simulink library "LiS_ECN_Model_lib"  (R2016a)
settings: Solver=ode45  StartTime=0.0  StopTime=10.0  RelTol=1e-3
undefined symbols (not defined in the file): C1_SOC_POLY20, C1_SOC_POLY30, C1_SOC_POLY50, C_man, Cap_all, DiscIntNeverNeededParam, OCV_POLYhigh20, OCV_POLYhigh30, OCV_POLYhigh50, OCV_POLYlow20, OCV_POLYlow30, OCV_POLYlow50, R1_SOC_POLY20, R1_SOC_POLY30, R1_SOC_POLY50, Ri_POLYhigh20, Ri_POLYhigh30, Ri_POLYhigh50, Ri_POLYlow20, Ri_POLYlow30, Ri_POLYlow50, StrechFactors, T, Tempstrech
libraries: simulink x1
settings Model: Creator=e102261  LastModifiedBy=e102261
settings DataIOCC: LimitDataPoints=on
settings DebuggingCC: AllowSymbolicDim=off

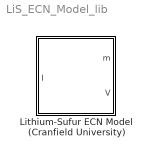
== system LiS_ECN_Model_lib ==
  Lithium-Sufur ECN Model (Cranfield University) : Subsystem  mask(Lithium-Sulfur ECN Model (Cranfield University)){TempDegC=21, InitialSoC=1, Ts=1}
      mask prompts: TempDegC "Temperature (degrees C):"; InitialSoC "Initial State-of-Charge (normalized):"; Ts "Sample time (-1 for inherited):"
      mask help:
      | This block contains an Equivalent Circuit (ECN) model of a representative lithium-sulfur cell supplied by OXIS Energy.  The model was developed as part of the Revolutionary Electric Vehicle Battery (REVB) project co-funded by Innovate UK, and contributions were made by people at Cranfield University, Imperial College London and OXIS Energy.
      |
      | This model is released in association with a the paper 'Multi-temperature state-dependent equivalent circuit discharge model for lithium-sulfur batteries' by Propp et al, accepted by the Journal of Power Sources on July 23, 2016, http://dx.doi.org/10.1016/j.jpowsour.2016.07.090.  Please reference this paper if you use this model.
      |
      | Please see the licence terms at http://dx.doi.org/10.17862/cranfield.rd.c.3292031
      mask init:
      | % Define the MATLAB data file.
      | MATLAB_DATA_FILE = 'LiS_ECN_Model_Parameters.mat';
      | 
      | % Check to see if the file exists: if not, fail gracefully.
      | fileExists = exist(MATLAB_DATA_FILE, 'file') > 0;
      | if ~fileExists
      |     id = 'LiS_ECN_Model:parameterFileNotFound';
      |     msg = {'Parameter file not found: %s.', MATLAB_DATA_FILE};
      |     ME = MException(id, msg{:});
      |     throw(ME);
      | end
      | 
      | % If the file does exist, then load it into the block
      | % workspace.
      | load(MATLAB_DATA_FILE);
      | 
      | try
      |     theImage = imread('oxiscellicon_simulink')
      | catch
      |     theImage = [];
      | end
      settings: AttributesFormatString=|
      | Temperature = %<TempDegC> deg C
      | Initial SoC = %<InitialSoC>
      mask Display:
      | patch([0 0 1 1],[0 1 1 0],[255 221 0]/255);
      | image(imread('oxis_li-s.png'),'center')
      | plot([0.5 0.5], [0.05 0.40]);
      | plot([0.35 0.35 0.65 0.65 0.35], [0.45 0.4 0.4 0.45 0.45]);
      | %patch([0.35 0.35 0.65 0.65 0.35], [0.45 0.4 0.4 0.45 0.45]);
      | plot([0.2 0.8], [0.55 0.55]);
      | plot([0.5 0.5], [0.55 0.95]);
      | 
      | port_label('output', 1, 'm')
      | color('blue')
      | port_label('input', 1, 'I(t)')
      | port_label('output', 2, 'V(t)')

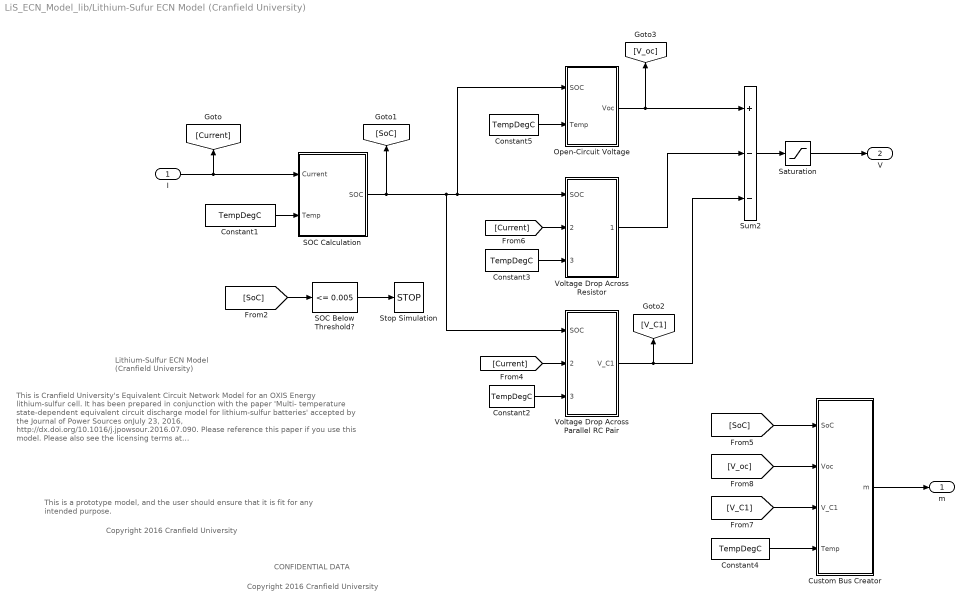
== system LiS_ECN_Model_lib/Lithium-Sufur ECN Model (Cranfield University) ==
  note: Copyright 2016 Cranfield University
  note: CONFIDENTIAL DATA
  note: Copyright 2016 Cranfield University
  note: This is Cranfield University's Equivalent Circuit Network Model for an OXIS Energy
      | lithium-sulfur cell. It has been prepared in conjunction with the paper 'Multi-
      | temperature state-dependent equivalent circuit discharge model for lithium-sulfur
      | batteries' accepted by the Journal of Power Sources onJuly 23, 2016,
      | http://dx.doi.org/10.1016/j.jpowsour.2016.07.090. Please reference this paper if
      | you use this model.
      |
      | Please also see the licensing terms at
      | http://dx.doi.org/10.17862/cranfield.rd.c.3292031
  note: Lithium-Sulfur ECN Model
      | (Cranfield University)
  note: This is a prototype model, and the user should ensure that it is fit for
      | any intended purpose.
  I : Inport  PortDimensions=1  SampleTime=Ts
      settings: AttributesFormatString=SampleTime=%<SampleTime>
  Constant{1..5} (5 alike) : Constant  Value=TempDegC
  Custom Bus Creator : Subsystem
  Open-Circuit Voltage : Subsystem
  SOC Below Threshold? : simulink/Logic and Bit Operations/Compare To Constant  relop=<=  const=0.005  OutDataTypeStr=boolean
  SOC Calculation : Subsystem
  Saturation : Saturate  UpperLimit=inf  LowerLimit=0
      settings: AttributesFormatString=|
      | UpperLimit=%<UpperLimit>
      | LowerLimit=%<LowerLimit>
  Stop Simulation : Stop
  Sum2 : Sum  Inputs=+--
  Voltage Drop Across Parallel RC Pair : Subsystem
  Voltage Drop Across Resistor : Subsystem
  m : Outport  SampleTime=Ts
      settings: AttributesFormatString=SampleTime=%<SampleTime>
  V : Outport  Port=2  SampleTime=Ts
      settings: AttributesFormatString=SampleTime=%<SampleTime>
  wires:
  Custom Bus Creator/1(m) -> m/1
  Constant4/1 -> Custom Bus Creator/4(Temp)
  [V_C1] -> Custom Bus Creator/3(V_C1)
  [V_oc] -> Custom Bus Creator/2(Voc)
  [SoC] -> Custom Bus Creator/1(SoC)
  SOC Below Threshold?/1 -> Stop Simulation/1
  Constant1/1 -> SOC Calculation/2(Temp)
  Constant2/1 -> Voltage Drop Across Parallel RC Pair/3(Temperature)
  Constant3/1 -> Voltage Drop Across Resistor/3(Temp)
  Constant5/1 -> Open-Circuit Voltage/2(Temp)
  Saturation/1 -> V/1
  SOC Calculation/1(SOC) -> [SoC], Voltage Drop Across Parallel RC Pair/1(SOC), Voltage Drop Across Resistor/1(SOC), Open-Circuit Voltage/1(SOC)
  [Current] -> Voltage Drop Across Parallel RC Pair/2(Current)
  Voltage Drop Across Parallel RC Pair/1(V_C1) -> [V_C1], Sum2/3
  Voltage Drop Across Resistor/1(V Rint) -> Sum2/2
  [Current] -> Voltage Drop Across Resistor/2(Current)
  Open-Circuit Voltage/1(Voc) -> [V_oc], Sum2/1
  [SoC] -> SOC Below Threshold?/1
  I/1 -> [Current], SOC Calculation/1(Current)
  Sum2/1 -> Saturation/1

== system LiS_ECN_Model_lib/Lithium-Sufur ECN Model (Cranfield University)/Custom Bus Creator ==
  SoC : Inport  PortDimensions=1  SampleTime=Ts
  Voc : Inport  Port=2  PortDimensions=1  SampleTime=Ts
  V_C1 : Inport  Port=3  PortDimensions=1  SampleTime=Ts
  Temp : Inport  Port=4  PortDimensions=1  SampleTime=Ts
  Bus Creator : BusCreator  Inputs=4
  m : Outport
  wires:
  Bus Creator/1 -> m/1
  Temp/1 -> Bus Creator/4  "Temperature (deg C)"
  V_C1/1 -> Bus Creator/3  "Voltage across C1 (V)"
  Voc/1 -> Bus Creator/2  "Open-circuit voltage (V)"
  SoC/1 -> Bus Creator/1  "State-of-Charge (dimensionless)"

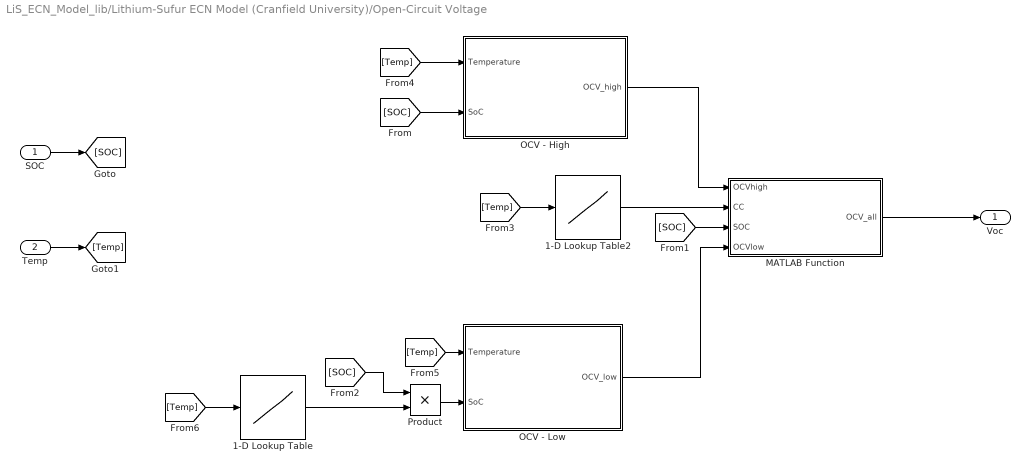
== system LiS_ECN_Model_lib/Lithium-Sufur ECN Model (Cranfield University)/Open-Circuit Voltage ==
  SOC : Inport
  Temp : Inport  Port=2
  1-D Lookup Table : Lookup_n-D  NumberOfTableDimensions=1  BreakpointsForDimension1=Tempstrech  Table=StrechFactors  InternalRulePriority=Speed  RndMeth=Simplest  InputSameDT=on
  1-D Lookup Table2 : Lookup_n-D  NumberOfTableDimensions=1  BreakpointsForDimension1=Temp'  Table=C_man  InternalRulePriority=Speed  RndMeth=Simplest  InputSameDT=on
  MATLAB Function : MATLAB Function  TreatAsAtomicUnit=on
  OCV - High : Subsystem
  OCV - Low : Subsystem
  Product : Product
  Voc : Outport
  wires:
  1-D Lookup Table2/1 -> MATLAB Function/2(CC)
  OCV - High/1("OCV_high ") -> MATLAB Function/1(OCVhigh)
  SOC/1 -> [SOC]
  [SOC] -> OCV - High/2(SoC)
  [SOC] -> MATLAB Function/3(SOC)
  [Temp] -> OCV - High/1(Temperature)
  [Temp] -> 1-D Lookup Table2/1
  [SOC] -> Product/1
  Temp/1 -> [Temp]
  [Temp] -> OCV - Low/1(Temperature)
  MATLAB Function/1(OCV_all) -> Voc/1
  [Temp] -> 1-D Lookup Table/1
  1-D Lookup Table/1 -> Product/2
  Product/1 -> OCV - Low/2(SoC)
  OCV - Low/1("OCV_low ") -> MATLAB Function/4(OCVlow)

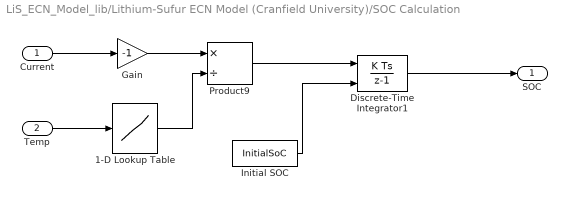
== system LiS_ECN_Model_lib/Lithium-Sufur ECN Model (Cranfield University)/SOC Calculation ==
  Current : Inport
  Temp : Inport  Port=2
  1-D Lookup Table : Lookup_n-D  NumberOfTableDimensions=1  BreakpointsForDimension1=T  Table=Cap_all  InternalRulePriority=Speed  RndMeth=Simplest  InputSameDT=on
  Discrete-Time Integrator1 : DiscreteIntegrator  InitialConditionSource=external  InitialConditionSetting=State (most efficient)  SampleTime=Ts  ICPrevOutput=DiscIntNeverNeededParam  ICPrevScaledInput=DiscIntNeverNeededParam
  Gain : Gain  Gain=-1
  Initial SOC : Constant  Value=InitialSoC
  Product9 : Product  Inputs=*/
  SOC : Outport
  wires:
  Initial SOC/1 -> Discrete-Time Integrator1/2
  Discrete-Time Integrator1/1 -> SOC/1
  1-D Lookup Table/1 -> Product9/2
  Temp/1 -> 1-D Lookup Table/1
  Product9/1 -> Discrete-Time Integrator1/1
  Gain/1 -> Product9/1
  Current/1 -> Gain/1

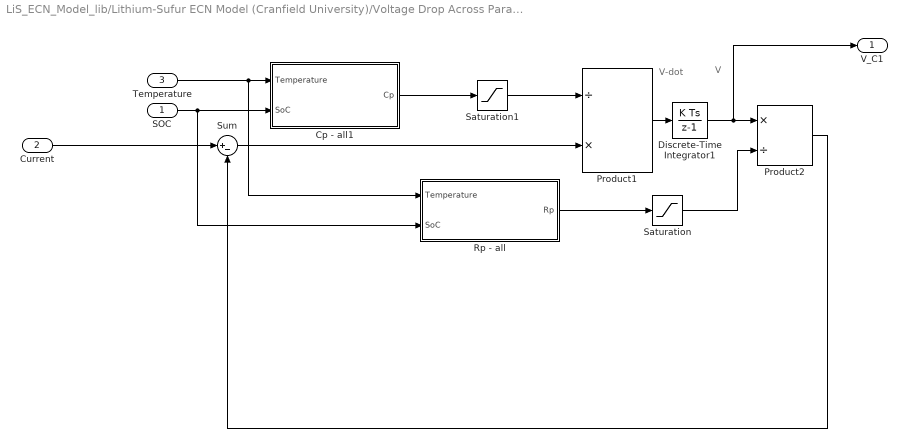
== system LiS_ECN_Model_lib/Lithium-Sufur ECN Model (Cranfield University)/Voltage Drop Across Parallel RC Pair ==
  note: V-dot
  note: V
  SOC : Inport
  Current : Inport  Port=2
  Temperature : Inport  Port=3
  Cp - all1 : Subsystem
  Discrete-Time Integrator1 : DiscreteIntegrator  SampleTime=Ts  ICPrevOutput=DiscIntNeverNeededParam  ICPrevScaledInput=DiscIntNeverNeededParam
  Product1 : Product  Inputs=/*
  Product2 : Product  Inputs=*/
  Rp - all : Subsystem
  Saturation : Saturate  UpperLimit=inf  LowerLimit=0.0001
  Saturation1 : Saturate  UpperLimit=50000  LowerLimit=10
  Sum : Sum  Inputs=|+-
  V_C1 : Outport
  wires:
  Temperature/1 -> Cp - all1/1(Temperature), Rp - all/1(Temperature)
  Cp - all1/1("Cp ") -> Saturation1/1
  Rp - all/1("Rp ") -> Saturation/1
  Product2/1 -> Sum/2
  Discrete-Time Integrator1/1 -> Product2/1, V_C1/1
  Saturation/1 -> Product2/2
  Product1/1 -> Discrete-Time Integrator1/1
  Sum/1 -> Product1/2
  Saturation1/1 -> Product1/1
  Current/1 -> Sum/1
  SOC/1 -> Cp - all1/2(SoC), Rp - all/2(SoC)

== system LiS_ECN_Model_lib/Lithium-Sufur ECN Model (Cranfield University)/Voltage Drop Across Resistor ==
  SOC : Inport
  Current : Inport  Port=2
  Temp : Inport  Port=3
  Product : Product
  Ri - All : Subsystem
  V Rint : Outport
  wires:
  Ri - All/1(Ri all) -> Product/1
  Temp/1 -> Ri - All/2(Temp1)
  SOC/1 -> Ri - All/1(SoC)
  Product/1 -> V Rint/1
  Current/1 -> Product/2

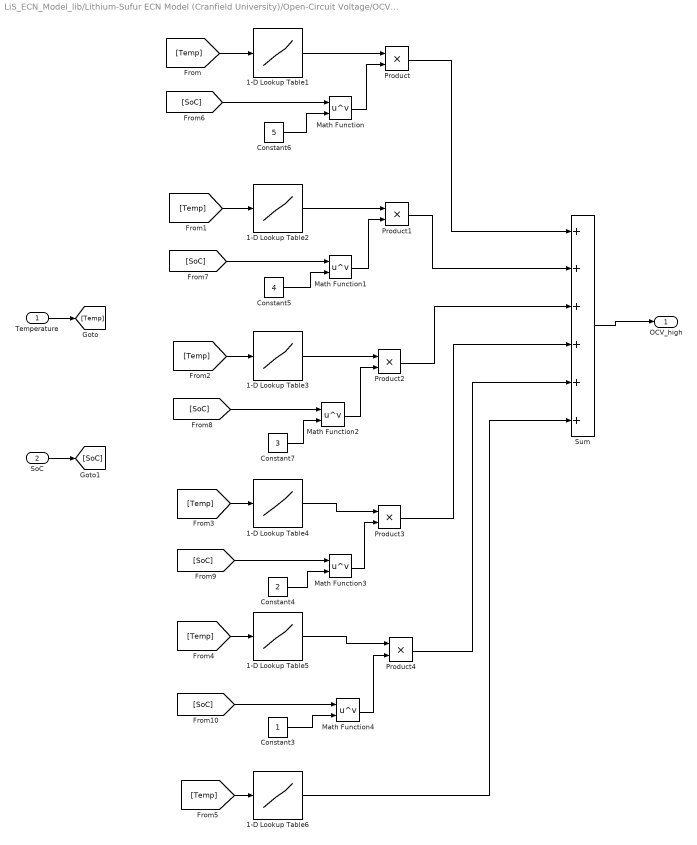
== system LiS_ECN_Model_lib/Lithium-Sufur ECN Model (Cranfield University)/Open-Circuit Voltage/OCV - High ==
  Temperature : Inport
  SoC : Inport  Port=2
  1-D Lookup Table1 : Lookup_n-D  NumberOfTableDimensions=1  BreakpointsForDimension1=T  Table=[OCV_POLYhigh20(1) ; OCV_POLYhigh30(1) ; OCV_POLYhigh50(1)]  InternalRulePriority=Speed  RndMeth=Simplest  InputSameDT=on
  1-D Lookup Table2 : Lookup_n-D  NumberOfTableDimensions=1  BreakpointsForDimension1=T  Table=[OCV_POLYhigh20(2) ; OCV_POLYhigh30(2) ; OCV_POLYhigh50(2)]  InternalRulePriority=Speed  RndMeth=Simplest  InputSameDT=on
  1-D Lookup Table3 : Lookup_n-D  NumberOfTableDimensions=1  BreakpointsForDimension1=T  Table=[OCV_POLYhigh20(3) ; OCV_POLYhigh30(3) ; OCV_POLYhigh50(3)]  InternalRulePriority=Speed  RndMeth=Simplest  InputSameDT=on
  1-D Lookup Table4 : Lookup_n-D  NumberOfTableDimensions=1  BreakpointsForDimension1=T  Table=[OCV_POLYhigh20(4) ; OCV_POLYhigh30(4) ; OCV_POLYhigh50(4)]  InternalRulePriority=Speed  RndMeth=Simplest  InputSameDT=on
  1-D Lookup Table5 : Lookup_n-D  NumberOfTableDimensions=1  BreakpointsForDimension1=T  Table=[OCV_POLYhigh20(5) ; OCV_POLYhigh30(5) ; OCV_POLYhigh50(5)]  InternalRulePriority=Speed  RndMeth=Simplest  InputSameDT=on
  1-D Lookup Table6 : Lookup_n-D  NumberOfTableDimensions=1  BreakpointsForDimension1=T  Table=[OCV_POLYhigh20(6) ; OCV_POLYhigh30(6) ; OCV_POLYhigh50(6)]  InternalRulePriority=Speed  RndMeth=Simplest  InputSameDT=on
  Constant3 : Constant
  Constant4 : Constant  Value=2
  Constant5 : Constant  Value=4
  Constant6 : Constant  Value=5
  Constant7 : Constant  Value=3
  Math Function{,1..4} (5 alike) : Math  Operator=pow  SaturateOnIntegerOverflow=on
  Product{,1..4} (5 alike) : Product
  Sum : Sum  Inputs=++++++
  "OCV_high " : Outport
  wires:
  SoC/1 -> [SoC]
  Constant6/1 -> Math Function/2
  Math Function4/1 -> Product4/2
  1-D Lookup Table4/1 -> Product3/1
  Math Function3/1 -> Product3/2
  Constant4/1 -> Math Function3/2
  Product2/1 -> Sum/3
  Product4/1 -> Sum/5
  1-D Lookup Table5/1 -> Product4/1
  Math Function2/1 -> Product2/2
  Product/1 -> Sum/1
  Constant7/1 -> Math Function2/2
  Product3/1 -> Sum/4
  Constant5/1 -> Math Function1/2
  1-D Lookup Table2/1 -> Product1/1
  Constant3/1 -> Math Function4/2
  1-D Lookup Table3/1 -> Product2/1
  1-D Lookup Table6/1 -> Sum/6
  Product1/1 -> Sum/2
  Math Function1/1 -> Product1/2
  1-D Lookup Table1/1 -> Product/1
  Math Function/1 -> Product/2
  [Temp] -> 1-D Lookup Table5/1
  [Temp] -> 1-D Lookup Table6/1
  [Temp] -> 1-D Lookup Table4/1
  [SoC] -> Math Function/1
  [SoC] -> Math Function2/1
  [SoC] -> Math Function4/1
  [SoC] -> Math Function3/1
  [SoC] -> Math Function1/1
  Temperature/1 -> [Temp]
  [Temp] -> 1-D Lookup Table1/1
  [Temp] -> 1-D Lookup Table2/1
  [Temp] -> 1-D Lookup Table3/1
  Sum/1 -> "OCV_high "/1

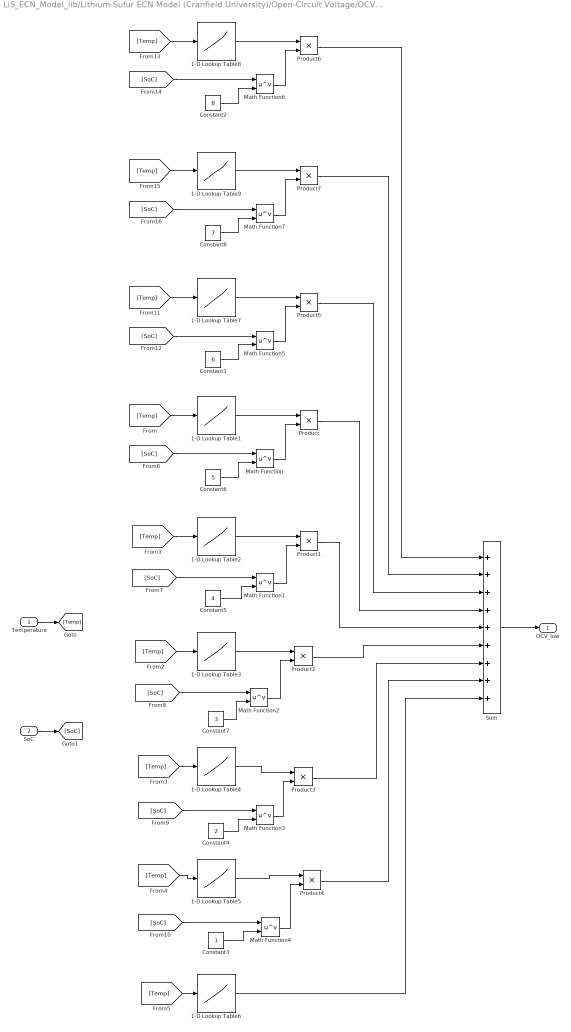
== system LiS_ECN_Model_lib/Lithium-Sufur ECN Model (Cranfield University)/Open-Circuit Voltage/OCV - Low ==
  Temperature : Inport
  SoC : Inport  Port=2
  1-D Lookup Table1 : Lookup_n-D  NumberOfTableDimensions=1  BreakpointsForDimension1=T  Table=[OCV_POLYlow20(4) ; OCV_POLYlow30(4) ; OCV_POLYlow50(4)]  InternalRulePriority=Speed  RndMeth=Simplest  InputSameDT=on
  1-D Lookup Table2 : Lookup_n-D  NumberOfTableDimensions=1  BreakpointsForDimension1=T  Table=[OCV_POLYlow20(5) ; OCV_POLYlow30(5) ; OCV_POLYlow50(5)]  InternalRulePriority=Speed  RndMeth=Simplest  InputSameDT=on
  1-D Lookup Table3 : Lookup_n-D  NumberOfTableDimensions=1  BreakpointsForDimension1=T  Table=[OCV_POLYlow20(6) ; OCV_POLYlow30(6) ; OCV_POLYlow50(6)]  InternalRulePriority=Speed  RndMeth=Simplest  InputSameDT=on
  1-D Lookup Table4 : Lookup_n-D  NumberOfTableDimensions=1  BreakpointsForDimension1=T  Table=[OCV_POLYlow20(7) ; OCV_POLYlow30(7) ; OCV_POLYlow50(7)]  InternalRulePriority=Speed  RndMeth=Simplest  InputSameDT=on
  1-D Lookup Table5 : Lookup_n-D  NumberOfTableDimensions=1  BreakpointsForDimension1=T  Table=[OCV_POLYlow20(8) ; OCV_POLYlow30(8) ; OCV_POLYlow50(8)]  InternalRulePriority=Speed  RndMeth=Simplest  InputSameDT=on
  1-D Lookup Table6 : Lookup_n-D  NumberOfTableDimensions=1  BreakpointsForDimension1=T  Table=[OCV_POLYlow20(9) ; OCV_POLYlow30(9) ; OCV_POLYlow50(9)]  InternalRulePriority=Speed  RndMeth=Simplest  InputSameDT=on
  1-D Lookup Table7 : Lookup_n-D  NumberOfTableDimensions=1  BreakpointsForDimension1=T  Table=[OCV_POLYlow20(3) ; OCV_POLYlow30(3) ; OCV_POLYlow50(3)]  InternalRulePriority=Speed  RndMeth=Simplest  InputSameDT=on
  1-D Lookup Table8 : Lookup_n-D  NumberOfTableDimensions=1  BreakpointsForDimension1=T  Table=[OCV_POLYlow20(1) ; OCV_POLYlow30(1) ; OCV_POLYlow50(1)]  InternalRulePriority=Speed  RndMeth=Simplest  InputSameDT=on
  1-D Lookup Table9 : Lookup_n-D  NumberOfTableDimensions=1  BreakpointsForDimension1=T  Table=[OCV_POLYlow20(2) ; OCV_POLYlow30(2) ; OCV_POLYlow50(2)]  InternalRulePriority=Speed  RndMeth=Simplest  InputSameDT=on
  Constant1 : Constant  Value=6
  Constant2 : Constant  Value=8
  Constant3 : Constant
  Constant4 : Constant  Value=2
  Constant5 : Constant  Value=4
  Constant6 : Constant  Value=5
  Constant7 : Constant  Value=3
  Constant8 : Constant  Value=7
  Math Function{,1..7} (8 alike) : Math  Operator=pow  SaturateOnIntegerOverflow=on
  Product{,1..7} (8 alike) : Product
  Sum : Sum  Inputs=+++++++++
  "OCV_low " : Outport
  wires:
  1-D Lookup Table6/1 -> Sum/9
  Product4/1 -> Sum/8
  Product3/1 -> Sum/7
  Product2/1 -> Sum/6
  Product1/1 -> Sum/5
  Product/1 -> Sum/4
  Product5/1 -> Sum/3
  Product7/1 -> Sum/2
  Product6/1 -> Sum/1
  Constant8/1 -> Math Function7/2
  1-D Lookup Table9/1 -> Product7/1
  Math Function7/1 -> Product7/2
  [SoC] -> Math Function7/1
  [Temp] -> 1-D Lookup Table9/1
  Constant2/1 -> Math Function6/2
  1-D Lookup Table8/1 -> Product6/1
  Math Function6/1 -> Product6/2
  [SoC] -> Math Function6/1
  [Temp] -> 1-D Lookup Table8/1
  Constant1/1 -> Math Function5/2
  1-D Lookup Table7/1 -> Product5/1
  Math Function5/1 -> Product5/2
  [SoC] -> Math Function5/1
  [Temp] -> 1-D Lookup Table7/1
  SoC/1 -> [SoC]
  Constant6/1 -> Math Function/2
  Math Function4/1 -> Product4/2
  1-D Lookup Table4/1 -> Product3/1
  Math Function3/1 -> Product3/2
  Constant4/1 -> Math Function3/2
  1-D Lookup Table5/1 -> Product4/1
  Math Function2/1 -> Product2/2
  Constant7/1 -> Math Function2/2
  Constant5/1 -> Math Function1/2
  1-D Lookup Table2/1 -> Product1/1
  Constant3/1 -> Math Function4/2
  1-D Lookup Table3/1 -> Product2/1
  Math Function1/1 -> Product1/2
  1-D Lookup Table1/1 -> Product/1
  Math Function/1 -> Product/2
  [Temp] -> 1-D Lookup Table5/1
  [Temp] -> 1-D Lookup Table6/1
  [Temp] -> 1-D Lookup Table4/1
  [SoC] -> Math Function/1
  [SoC] -> Math Function2/1
  [SoC] -> Math Function4/1
  [SoC] -> Math Function3/1
  [SoC] -> Math Function1/1
  Temperature/1 -> [Temp]
  [Temp] -> 1-D Lookup Table1/1
  [Temp] -> 1-D Lookup Table2/1
  [Temp] -> 1-D Lookup Table3/1
  Sum/1 -> "OCV_low "/1

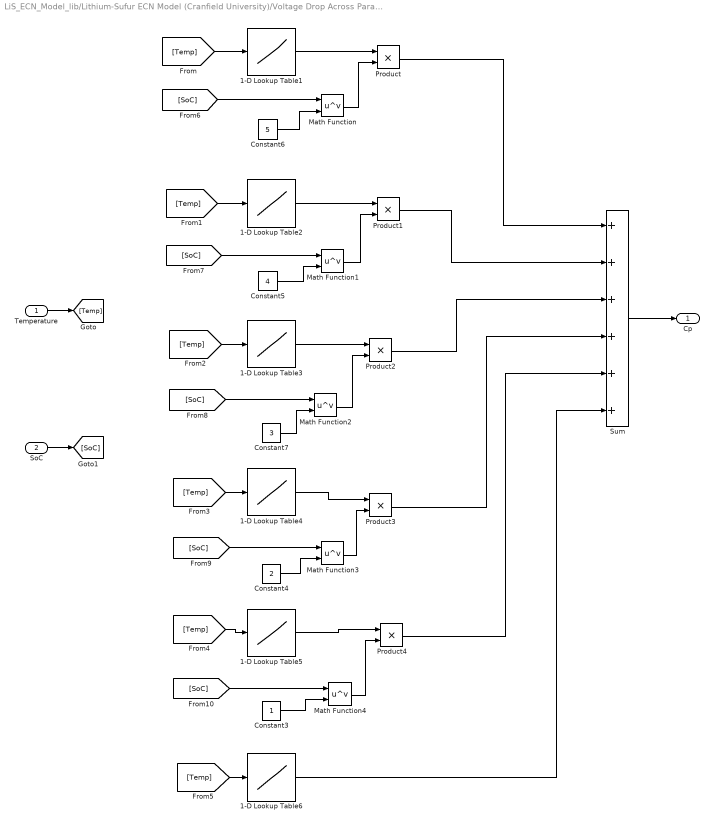
== system LiS_ECN_Model_lib/Lithium-Sufur ECN Model (Cranfield University)/Voltage Drop Across Parallel RC Pair/Cp - all1 ==
  Temperature : Inport
  SoC : Inport  Port=2
  1-D Lookup Table1 : Lookup_n-D  NumberOfTableDimensions=1  BreakpointsForDimension1=T  Table=[C1_SOC_POLY20(1) ; C1_SOC_POLY30(1) ; C1_SOC_POLY50(1)]  InternalRulePriority=Speed  RndMeth=Simplest  InputSameDT=on
  1-D Lookup Table2 : Lookup_n-D  NumberOfTableDimensions=1  BreakpointsForDimension1=T  Table=[C1_SOC_POLY20(2) ; C1_SOC_POLY30(2) ; C1_SOC_POLY50(2)]  InternalRulePriority=Speed  RndMeth=Simplest  InputSameDT=on
  1-D Lookup Table3 : Lookup_n-D  NumberOfTableDimensions=1  BreakpointsForDimension1=T  Table=[C1_SOC_POLY20(3) ; C1_SOC_POLY30(3) ; C1_SOC_POLY50(3)]  InternalRulePriority=Speed  RndMeth=Simplest  InputSameDT=on
  1-D Lookup Table4 : Lookup_n-D  NumberOfTableDimensions=1  BreakpointsForDimension1=T  Table=[C1_SOC_POLY20(4) ; C1_SOC_POLY30(4) ; C1_SOC_POLY50(4)]  InternalRulePriority=Speed  RndMeth=Simplest  InputSameDT=on
  1-D Lookup Table5 : Lookup_n-D  NumberOfTableDimensions=1  BreakpointsForDimension1=T  Table=[C1_SOC_POLY20(5) ; C1_SOC_POLY30(5) ; C1_SOC_POLY50(5)]  InternalRulePriority=Speed  RndMeth=Simplest  InputSameDT=on
  1-D Lookup Table6 : Lookup_n-D  NumberOfTableDimensions=1  BreakpointsForDimension1=T  Table=[C1_SOC_POLY20(6) ; C1_SOC_POLY30(6) ; C1_SOC_POLY50(6)]  InternalRulePriority=Speed  RndMeth=Simplest  InputSameDT=on
  Constant3 : Constant
  Constant4 : Constant  Value=2
  Constant5 : Constant  Value=4
  Constant6 : Constant  Value=5
  Constant7 : Constant  Value=3
  Math Function{,1..4} (5 alike) : Math  Operator=pow  SaturateOnIntegerOverflow=on
  Product{,1..4} (5 alike) : Product
  Sum : Sum  Inputs=++++++
  "Cp " : Outport
  wires:
  1-D Lookup Table6/1 -> Sum/6
  Product4/1 -> Sum/5
  Product3/1 -> Sum/4
  Product2/1 -> Sum/3
  Product1/1 -> Sum/2
  Product/1 -> Sum/1
  SoC/1 -> [SoC]
  Constant6/1 -> Math Function/2
  Math Function4/1 -> Product4/2
  1-D Lookup Table4/1 -> Product3/1
  Math Function3/1 -> Product3/2
  Constant4/1 -> Math Function3/2
  1-D Lookup Table5/1 -> Product4/1
  Math Function2/1 -> Product2/2
  Constant7/1 -> Math Function2/2
  Constant5/1 -> Math Function1/2
  1-D Lookup Table2/1 -> Product1/1
  Constant3/1 -> Math Function4/2
  1-D Lookup Table3/1 -> Product2/1
  Math Function1/1 -> Product1/2
  1-D Lookup Table1/1 -> Product/1
  Math Function/1 -> Product/2
  [Temp] -> 1-D Lookup Table5/1
  [Temp] -> 1-D Lookup Table6/1
  [Temp] -> 1-D Lookup Table4/1
  [SoC] -> Math Function/1
  [SoC] -> Math Function2/1
  [SoC] -> Math Function4/1
  [SoC] -> Math Function3/1
  [SoC] -> Math Function1/1
  Temperature/1 -> [Temp]
  [Temp] -> 1-D Lookup Table1/1
  [Temp] -> 1-D Lookup Table2/1
  [Temp] -> 1-D Lookup Table3/1
  Sum/1 -> "Cp "/1

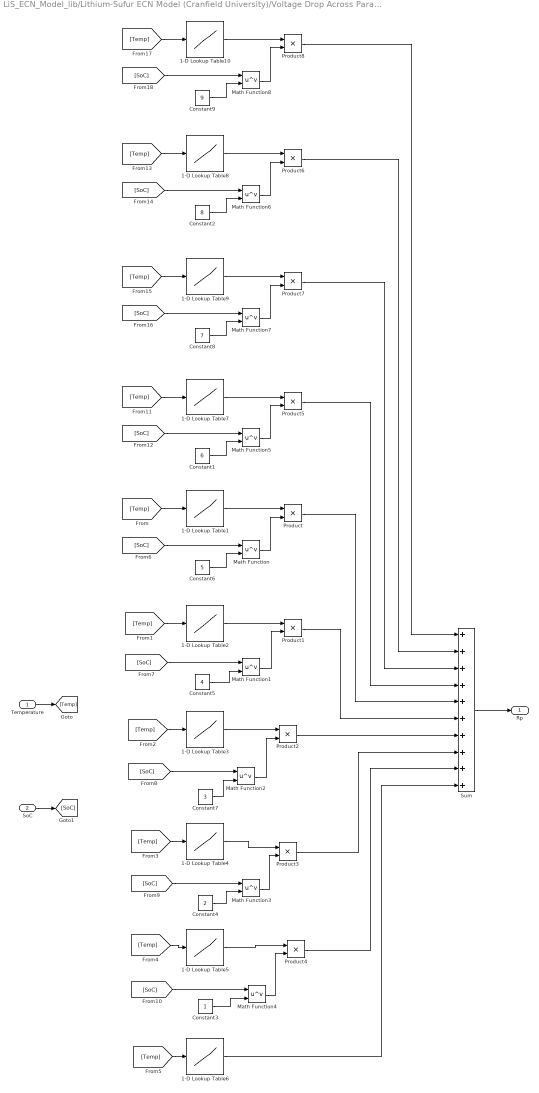
== system LiS_ECN_Model_lib/Lithium-Sufur ECN Model (Cranfield University)/Voltage Drop Across Parallel RC Pair/Rp - all ==
  Temperature : Inport
  SoC : Inport  Port=2
  1-D Lookup Table1 : Lookup_n-D  NumberOfTableDimensions=1  BreakpointsForDimension1=T  Table=[R1_SOC_POLY20(5) ; R1_SOC_POLY30(5) ; R1_SOC_POLY50(5)]  InternalRulePriority=Speed  RndMeth=Simplest  InputSameDT=on
  1-D Lookup Table10 : Lookup_n-D  NumberOfTableDimensions=1  BreakpointsForDimension1=T  Table=[R1_SOC_POLY20(1) ; R1_SOC_POLY30(1) ; R1_SOC_POLY50(1)]  InternalRulePriority=Speed  RndMeth=Simplest  InputSameDT=on
  1-D Lookup Table2 : Lookup_n-D  NumberOfTableDimensions=1  BreakpointsForDimension1=T  Table=[R1_SOC_POLY20(6) ; R1_SOC_POLY30(6) ; R1_SOC_POLY50(6)]  InternalRulePriority=Speed  RndMeth=Simplest  InputSameDT=on
  1-D Lookup Table3 : Lookup_n-D  NumberOfTableDimensions=1  BreakpointsForDimension1=T  Table=[R1_SOC_POLY20(7) ; R1_SOC_POLY30(7) ; R1_SOC_POLY50(7)]  InternalRulePriority=Speed  RndMeth=Simplest  InputSameDT=on
  1-D Lookup Table4 : Lookup_n-D  NumberOfTableDimensions=1  BreakpointsForDimension1=T  Table=[R1_SOC_POLY20(8) ; R1_SOC_POLY30(8) ; R1_SOC_POLY50(8)]  InternalRulePriority=Speed  RndMeth=Simplest  InputSameDT=on
  1-D Lookup Table5 : Lookup_n-D  NumberOfTableDimensions=1  BreakpointsForDimension1=T  Table=[R1_SOC_POLY20(9) ; R1_SOC_POLY30(9) ; R1_SOC_POLY50(9)]  InternalRulePriority=Speed  RndMeth=Simplest  InputSameDT=on
  1-D Lookup Table6 : Lookup_n-D  NumberOfTableDimensions=1  BreakpointsForDimension1=T  Table=[R1_SOC_POLY20(10) ; R1_SOC_POLY30(10) ; R1_SOC_POLY50(10)]  InternalRulePriority=Speed  RndMeth=Simplest  InputSameDT=on
  1-D Lookup Table7 : Lookup_n-D  NumberOfTableDimensions=1  BreakpointsForDimension1=T  Table=[R1_SOC_POLY20(4) ; R1_SOC_POLY30(4) ; R1_SOC_POLY50(4)]  InternalRulePriority=Speed  RndMeth=Simplest  InputSameDT=on
  1-D Lookup Table8 : Lookup_n-D  NumberOfTableDimensions=1  BreakpointsForDimension1=T  Table=[R1_SOC_POLY20(2) ; R1_SOC_POLY30(2) ; R1_SOC_POLY50(2)]  InternalRulePriority=Speed  RndMeth=Simplest  InputSameDT=on
  1-D Lookup Table9 : Lookup_n-D  NumberOfTableDimensions=1  BreakpointsForDimension1=T  Table=[R1_SOC_POLY20(3) ; R1_SOC_POLY30(3) ; R1_SOC_POLY50(3)]  InternalRulePriority=Speed  RndMeth=Simplest  InputSameDT=on
  Constant1 : Constant  Value=6
  Constant2 : Constant  Value=8
  Constant3 : Constant
  Constant4 : Constant  Value=2
  Constant5 : Constant  Value=4
  Constant6 : Constant  Value=5
  Constant7 : Constant  Value=3
  Constant8 : Constant  Value=7
  Constant9 : Constant  Value=9
  Math Function{,1..8} (9 alike) : Math  Operator=pow  SaturateOnIntegerOverflow=on
  Product{,1..8} (9 alike) : Product
  Sum : Sum  Inputs=++++++++++
  "Rp " : Outport
  wires:
  Product8/1 -> Sum/1
  Product6/1 -> Sum/2
  Product7/1 -> Sum/3
  Product5/1 -> Sum/4
  Product/1 -> Sum/5
  Product1/1 -> Sum/6
  Product2/1 -> Sum/7
  Product3/1 -> Sum/8
  Product4/1 -> Sum/9
  1-D Lookup Table6/1 -> Sum/10
  Constant9/1 -> Math Function8/2
  1-D Lookup Table10/1 -> Product8/1
  Math Function8/1 -> Product8/2
  [SoC] -> Math Function8/1
  [Temp] -> 1-D Lookup Table10/1
  Constant8/1 -> Math Function7/2
  1-D Lookup Table9/1 -> Product7/1
  Math Function7/1 -> Product7/2
  [SoC] -> Math Function7/1
  [Temp] -> 1-D Lookup Table9/1
  Constant2/1 -> Math Function6/2
  1-D Lookup Table8/1 -> Product6/1
  Math Function6/1 -> Product6/2
  [SoC] -> Math Function6/1
  [Temp] -> 1-D Lookup Table8/1
  Constant1/1 -> Math Function5/2
  1-D Lookup Table7/1 -> Product5/1
  Math Function5/1 -> Product5/2
  [SoC] -> Math Function5/1
  [Temp] -> 1-D Lookup Table7/1
  SoC/1 -> [SoC]
  Constant6/1 -> Math Function/2
  Math Function4/1 -> Product4/2
  1-D Lookup Table4/1 -> Product3/1
  Math Function3/1 -> Product3/2
  Constant4/1 -> Math Function3/2
  1-D Lookup Table5/1 -> Product4/1
  Math Function2/1 -> Product2/2
  Constant7/1 -> Math Function2/2
  Constant5/1 -> Math Function1/2
  1-D Lookup Table2/1 -> Product1/1
  Constant3/1 -> Math Function4/2
  1-D Lookup Table3/1 -> Product2/1
  Math Function1/1 -> Product1/2
  1-D Lookup Table1/1 -> Product/1
  Math Function/1 -> Product/2
  [Temp] -> 1-D Lookup Table5/1
  [Temp] -> 1-D Lookup Table6/1
  [Temp] -> 1-D Lookup Table4/1
  [SoC] -> Math Function/1
  [SoC] -> Math Function2/1
  [SoC] -> Math Function4/1
  [SoC] -> Math Function3/1
  [SoC] -> Math Function1/1
  Temperature/1 -> [Temp]
  [Temp] -> 1-D Lookup Table1/1
  [Temp] -> 1-D Lookup Table2/1
  [Temp] -> 1-D Lookup Table3/1
  Sum/1 -> "Rp "/1

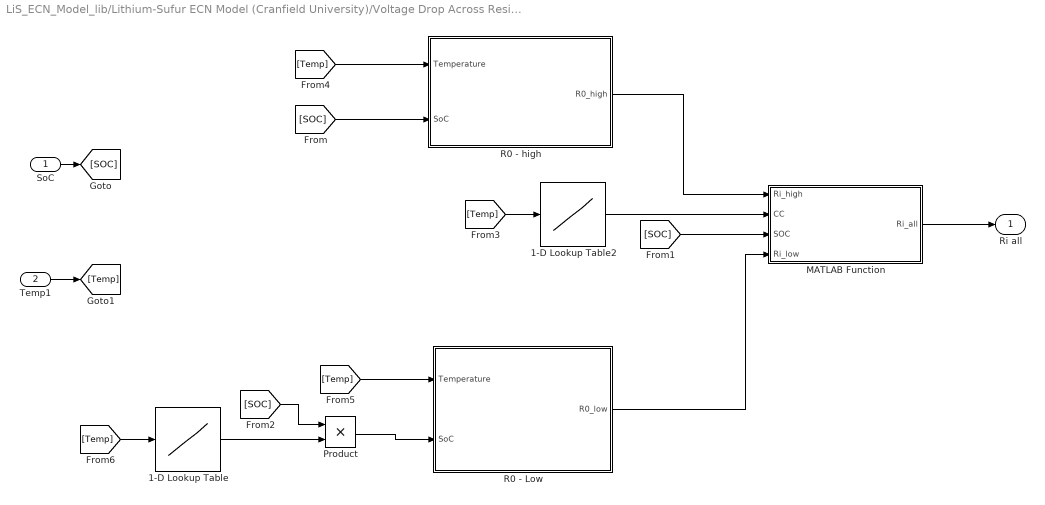
== system LiS_ECN_Model_lib/Lithium-Sufur ECN Model (Cranfield University)/Voltage Drop Across Resistor/Ri - All ==
  SoC : Inport
  Temp1 : Inport  Port=2
  1-D Lookup Table : Lookup_n-D  NumberOfTableDimensions=1  BreakpointsForDimension1=Tempstrech  Table=StrechFactors  InternalRulePriority=Speed  RndMeth=Simplest  InputSameDT=on
  1-D Lookup Table2 : Lookup_n-D  NumberOfTableDimensions=1  BreakpointsForDimension1=Temp'  Table=C_man  InternalRulePriority=Speed  RndMeth=Simplest  InputSameDT=on
  MATLAB Function : MATLAB Function  TreatAsAtomicUnit=on
  Product : Product
  R0 - Low : Subsystem
  R0 - high : Subsystem
  Ri all : Outport
  wires:
  [SOC] -> MATLAB Function/3(SOC)
  1-D Lookup Table2/1 -> MATLAB Function/2(CC)
  [Temp] -> 1-D Lookup Table2/1
  R0 - high/1("R0_high ") -> MATLAB Function/1(Ri_high)
  R0 - Low/1("R0_low ") -> MATLAB Function/4(Ri_low)
  MATLAB Function/1(Ri_all) -> Ri all/1
  [SOC] -> R0 - high/2(SoC)
  [SOC] -> Product/1
  [Temp] -> R0 - high/1(Temperature)
  Product/1 -> R0 - Low/2(SoC)
  1-D Lookup Table/1 -> Product/2
  [Temp] -> 1-D Lookup Table/1
  [Temp] -> R0 - Low/1(Temperature)
  SoC/1 -> [SOC]
  Temp1/1 -> [Temp]

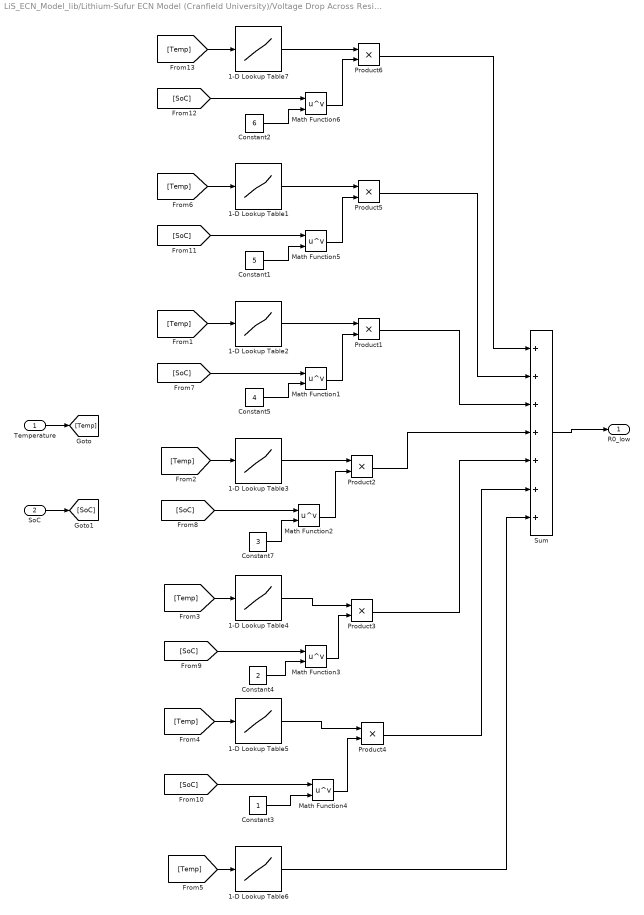
== system LiS_ECN_Model_lib/Lithium-Sufur ECN Model (Cranfield University)/Voltage Drop Across Resistor/Ri - All/R0 - Low ==
  Temperature : Inport
  SoC : Inport  Port=2
  1-D Lookup Table1 : Lookup_n-D  NumberOfTableDimensions=1  BreakpointsForDimension1=T  Table=[Ri_POLYlow20(2) ; Ri_POLYlow30(2) ; Ri_POLYlow50(2)]  InternalRulePriority=Speed  RndMeth=Simplest  InputSameDT=on
  1-D Lookup Table2 : Lookup_n-D  NumberOfTableDimensions=1  BreakpointsForDimension1=T  Table=[Ri_POLYlow20(3) ; Ri_POLYlow30(3) ; Ri_POLYlow50(3)]  InternalRulePriority=Speed  RndMeth=Simplest  InputSameDT=on
  1-D Lookup Table3 : Lookup_n-D  NumberOfTableDimensions=1  BreakpointsForDimension1=T  Table=[Ri_POLYlow20(4) ; Ri_POLYlow30(4) ; Ri_POLYlow50(4)]  InternalRulePriority=Speed  RndMeth=Simplest  InputSameDT=on
  1-D Lookup Table4 : Lookup_n-D  NumberOfTableDimensions=1  BreakpointsForDimension1=T  Table=[Ri_POLYlow20(5) ; Ri_POLYlow30(5) ; Ri_POLYlow50(5)]  InternalRulePriority=Speed  RndMeth=Simplest  InputSameDT=on
  1-D Lookup Table5 : Lookup_n-D  NumberOfTableDimensions=1  BreakpointsForDimension1=T  Table=[Ri_POLYlow20(6) ; Ri_POLYlow30(6) ; Ri_POLYlow50(6)]  InternalRulePriority=Speed  RndMeth=Simplest  InputSameDT=on
  1-D Lookup Table6 : Lookup_n-D  NumberOfTableDimensions=1  BreakpointsForDimension1=T  Table=[Ri_POLYlow20(7) ; Ri_POLYlow30(7) ; Ri_POLYlow50(7)]  InternalRulePriority=Speed  RndMeth=Simplest  InputSameDT=on
  1-D Lookup Table7 : Lookup_n-D  NumberOfTableDimensions=1  BreakpointsForDimension1=T  Table=[Ri_POLYlow20(1) ; Ri_POLYlow30(1) ; Ri_POLYlow50(1)]  InternalRulePriority=Speed  RndMeth=Simplest  InputSameDT=on
  Constant1 : Constant  Value=5
  Constant2 : Constant  Value=6
  Constant3 : Constant
  Constant4 : Constant  Value=2
  Constant5 : Constant  Value=4
  Constant7 : Constant  Value=3
  Math Function{1..6} (6 alike) : Math  Operator=pow  SaturateOnIntegerOverflow=on
  Product{1..6} (6 alike) : Product
  Sum : Sum  Inputs=+++++++
  "R0_low " : Outport
  wires:
  1-D Lookup Table6/1 -> Sum/7
  Product4/1 -> Sum/6
  Product3/1 -> Sum/5
  Product2/1 -> Sum/4
  Product1/1 -> Sum/3
  Product5/1 -> Sum/2
  Product6/1 -> Sum/1
  Constant2/1 -> Math Function6/2
  1-D Lookup Table7/1 -> Product6/1
  Math Function6/1 -> Product6/2
  [SoC] -> Math Function6/1
  [Temp] -> 1-D Lookup Table7/1
  Constant1/1 -> Math Function5/2
  1-D Lookup Table1/1 -> Product5/1
  Math Function5/1 -> Product5/2
  [SoC] -> Math Function5/1
  [Temp] -> 1-D Lookup Table1/1
  SoC/1 -> [SoC]
  Math Function4/1 -> Product4/2
  1-D Lookup Table4/1 -> Product3/1
  Math Function3/1 -> Product3/2
  Constant4/1 -> Math Function3/2
  1-D Lookup Table5/1 -> Product4/1
  Math Function2/1 -> Product2/2
  Constant7/1 -> Math Function2/2
  Constant5/1 -> Math Function1/2
  1-D Lookup Table2/1 -> Product1/1
  Constant3/1 -> Math Function4/2
  1-D Lookup Table3/1 -> Product2/1
  Math Function1/1 -> Product1/2
  [Temp] -> 1-D Lookup Table5/1
  [Temp] -> 1-D Lookup Table6/1
  [Temp] -> 1-D Lookup Table4/1
  [SoC] -> Math Function2/1
  [SoC] -> Math Function4/1
  [SoC] -> Math Function3/1
  [SoC] -> Math Function1/1
  Temperature/1 -> [Temp]
  [Temp] -> 1-D Lookup Table2/1
  [Temp] -> 1-D Lookup Table3/1
  Sum/1 -> "R0_low "/1

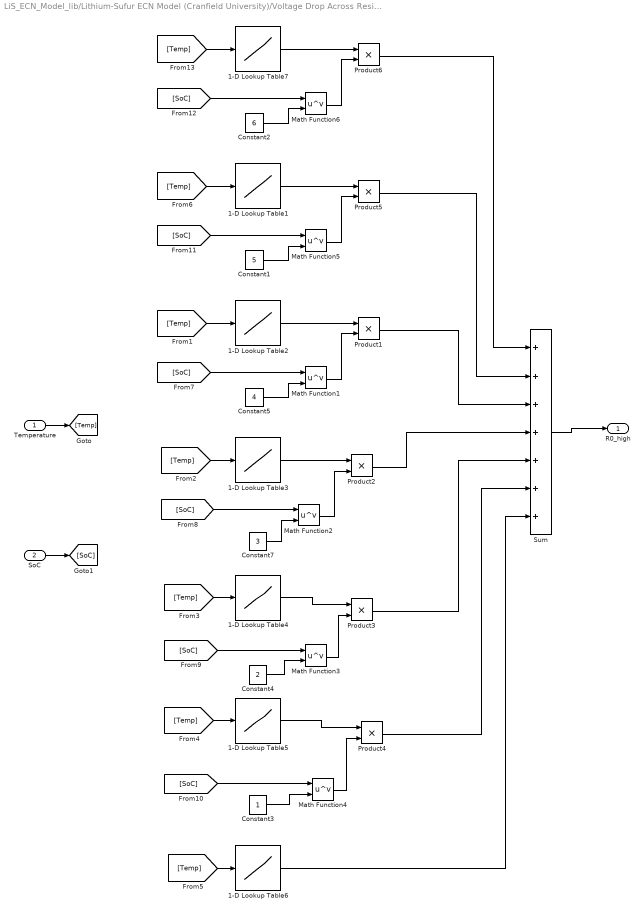
== system LiS_ECN_Model_lib/Lithium-Sufur ECN Model (Cranfield University)/Voltage Drop Across Resistor/Ri - All/R0 - high ==
  Temperature : Inport
  SoC : Inport  Port=2
  1-D Lookup Table1 : Lookup_n-D  NumberOfTableDimensions=1  BreakpointsForDimension1=T  Table=[Ri_POLYhigh20(2) ; Ri_POLYhigh30(2) ; Ri_POLYhigh50(2)]  InternalRulePriority=Speed  RndMeth=Simplest  InputSameDT=on
  1-D Lookup Table2 : Lookup_n-D  NumberOfTableDimensions=1  BreakpointsForDimension1=T  Table=[Ri_POLYhigh20(3) ; Ri_POLYhigh30(3) ; Ri_POLYhigh50(3)]  InternalRulePriority=Speed  RndMeth=Simplest  InputSameDT=on
  1-D Lookup Table3 : Lookup_n-D  NumberOfTableDimensions=1  BreakpointsForDimension1=T  Table=[Ri_POLYhigh20(4) ; Ri_POLYhigh30(4) ; Ri_POLYhigh50(4)]  InternalRulePriority=Speed  RndMeth=Simplest  InputSameDT=on
  1-D Lookup Table4 : Lookup_n-D  NumberOfTableDimensions=1  BreakpointsForDimension1=T  Table=[Ri_POLYhigh20(5) ; Ri_POLYhigh30(5) ; Ri_POLYhigh50(5)]  InternalRulePriority=Speed  RndMeth=Simplest  InputSameDT=on
  1-D Lookup Table5 : Lookup_n-D  NumberOfTableDimensions=1  BreakpointsForDimension1=T  Table=[Ri_POLYhigh20(6) ; Ri_POLYhigh30(6) ; Ri_POLYhigh50(6)]  InternalRulePriority=Speed  RndMeth=Simplest  InputSameDT=on
  1-D Lookup Table6 : Lookup_n-D  NumberOfTableDimensions=1  BreakpointsForDimension1=T  Table=[Ri_POLYhigh20(7) ; Ri_POLYhigh30(7) ; Ri_POLYhigh50(7)]  InternalRulePriority=Speed  RndMeth=Simplest  InputSameDT=on
  1-D Lookup Table7 : Lookup_n-D  NumberOfTableDimensions=1  BreakpointsForDimension1=T  Table=[Ri_POLYhigh20(1) ; Ri_POLYhigh30(1) ; Ri_POLYhigh50(1)]  InternalRulePriority=Speed  RndMeth=Simplest  InputSameDT=on
  Constant1 : Constant  Value=5
  Constant2 : Constant  Value=6
  Constant3 : Constant
  Constant4 : Constant  Value=2
  Constant5 : Constant  Value=4
  Constant7 : Constant  Value=3
  Math Function{1..6} (6 alike) : Math  Operator=pow  SaturateOnIntegerOverflow=on
  Product{1..6} (6 alike) : Product
  Sum : Sum  Inputs=+++++++
  "R0_high " : Outport
  wires:
  1-D Lookup Table6/1 -> Sum/7
  Product4/1 -> Sum/6
  Product3/1 -> Sum/5
  Product2/1 -> Sum/4
  Product1/1 -> Sum/3
  Product5/1 -> Sum/2
  Product6/1 -> Sum/1
  Constant2/1 -> Math Function6/2
  1-D Lookup Table7/1 -> Product6/1
  Math Function6/1 -> Product6/2
  [SoC] -> Math Function6/1
  [Temp] -> 1-D Lookup Table7/1
  Constant1/1 -> Math Function5/2
  1-D Lookup Table1/1 -> Product5/1
  Math Function5/1 -> Product5/2
  [SoC] -> Math Function5/1
  [Temp] -> 1-D Lookup Table1/1
  SoC/1 -> [SoC]
  Math Function4/1 -> Product4/2
  1-D Lookup Table4/1 -> Product3/1
  Math Function3/1 -> Product3/2
  Constant4/1 -> Math Function3/2
  1-D Lookup Table5/1 -> Product4/1
  Math Function2/1 -> Product2/2
  Constant7/1 -> Math Function2/2
  Constant5/1 -> Math Function1/2
  1-D Lookup Table2/1 -> Product1/1
  Constant3/1 -> Math Function4/2
  1-D Lookup Table3/1 -> Product2/1
  Math Function1/1 -> Product1/2
  [Temp] -> 1-D Lookup Table5/1
  [Temp] -> 1-D Lookup Table6/1
  [Temp] -> 1-D Lookup Table4/1
  [SoC] -> Math Function2/1
  [SoC] -> Math Function4/1
  [SoC] -> Math Function3/1
  [SoC] -> Math Function1/1
  Temperature/1 -> [Temp]
  [Temp] -> 1-D Lookup Table2/1
  [Temp] -> 1-D Lookup Table3/1
  Sum/1 -> "R0_high "/1

== matlab function LiS_ECN_Model_lib/Lithium-Sufur ECN Model (Cranfield University)/Voltage Drop Across Resistor/Ri - All/MATLAB Function ==
  data: Ri_high input; CC input; SOC input; Ri_all output; Ri_low input
function Ri_all = OCV_all(Ri_high, CC, SOC, Ri_low )
%#codegen

insin = 2*50*(SOC-CC);
gamma1 = 0.5 + 0.5*sin(insin);

if insin < -0.5*pi()
    test2 = 0;
elseif (-0.5*pi() <= insin) && (insin < 0.5*pi() )
    test2 = gamma1;
else
    test2 = 1;
end


    
Ri_all  = (1-test2) * Ri_low + test2 * Ri_high;

== matlab function LiS_ECN_Model_lib/Lithium-Sufur ECN Model (Cranfield University)/Open-Circuit Voltage/MATLAB Function ==
  data: OCVhigh input; CC input; SOC input; OCV_all output; OCVlow input
function OCV_all = OCV_all(OCVhigh, CC, SOC, OCVlow )
%#codegen

insin = 2*50*(SOC-CC);
gamma1 = 0.5 + 0.5*sin(insin);
    
if insin < -0.5*pi()
    test2 = 0;
elseif (-0.5*pi() <= insin) && (insin < 0.5*pi()) 
    test2 = gamma1;
else % if (insin > 0.5*pi() )
    test2 = 1;
end

OCV_all = (1-test2) * OCVlow + test2 * OCVhigh;
